simulink library "csc_sqt_sequential_trigger_mtv_lib"  (R2014b)
settings: Solver=ode45  SolverMode=SingleTasking  StartTime=0.0  StopTime=10.0  RelTol=1e-3
libraries: util_info_lib x1, csc_fcv_filter_convergence_lib x1, csc_squ_sequential_update_lib x1, csu_mmh_measurement_model_mtv_lib x1
settings Model: ExtModeAutoUpdateStatusClock=off  Creator=escrane  LastModifiedBy=mstewart

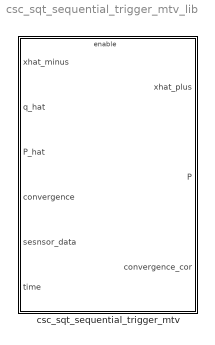
== system csc_sqt_sequential_trigger_mtv_lib ==
  csc_sqt_sequential_trigger_mtv : Subsystem  TreatAsAtomicUnit=on

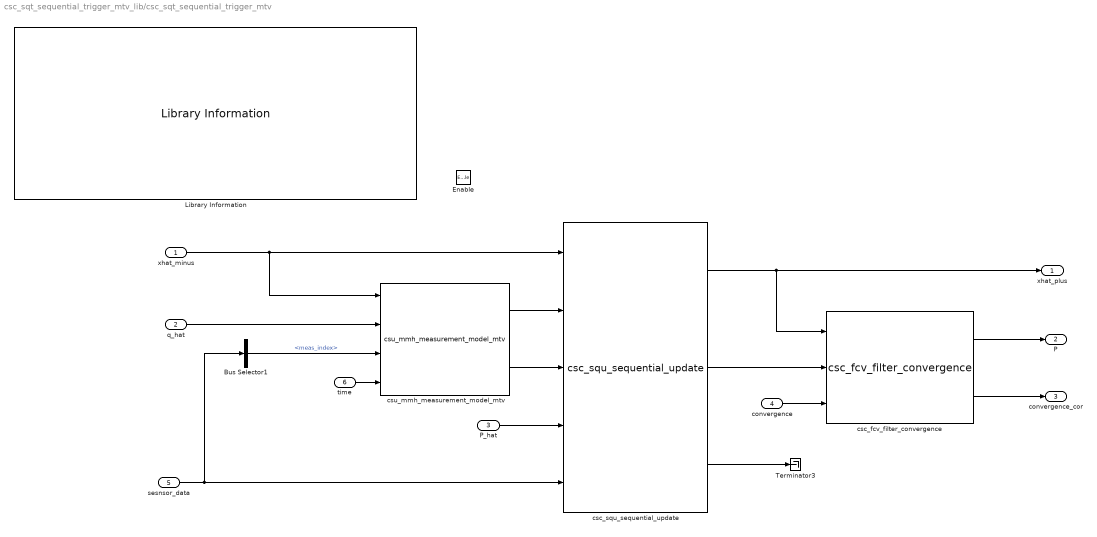
== system csc_sqt_sequential_trigger_mtv_lib/csc_sqt_sequential_trigger_mtv ==
  xhat_minus : Inport
  q_hat : Inport  Port=2
  P_hat : Inport  Port=3
  convergence : Inport  Port=4
  sesnsor_data : Inport  Port=5
  time : Inport  Port=6
  Enable : EnablePort
  Bus Selector1 : BusSelector  OutputSignals=meas_index
  Library Information : util_info_lib/Library Information  owner='NONE'
  Terminator3 : Terminator
  csc_fcv_filter_convergence : csc_fcv_filter_convergence_lib/csc_fcv_filter_convergence
  csc_squ_sequential_update : csc_squ_sequential_update_lib/csc_squ_sequential_update
  csu_mmh_measurement_model_mtv : csu_mmh_measurement_model_mtv_lib/csu_mmh_measurement_model_mtv
  xhat_plus : Outport
  P : Outport  Port=2
  convergence_cor : Outport  Port=3
  wires:
  convergence/1 -> csc_fcv_filter_convergence/3
  csc_squ_sequential_update/2 -> csc_fcv_filter_convergence/2
  csc_fcv_filter_convergence/2 -> convergence_cor/1
  csc_fcv_filter_convergence/1 -> P/1
  csc_squ_sequential_update/3 -> Terminator3/1
  time/1 -> csu_mmh_measurement_model_mtv/4
  csu_mmh_measurement_model_mtv/1 -> csc_squ_sequential_update/2
  Bus Selector1/1 -> csu_mmh_measurement_model_mtv/3  "<meas_index>"
  q_hat/1 -> csu_mmh_measurement_model_mtv/2
  csu_mmh_measurement_model_mtv/2 -> csc_squ_sequential_update/3
  xhat_minus/1 -> csc_squ_sequential_update/1, csu_mmh_measurement_model_mtv/1
  P_hat/1 -> csc_squ_sequential_update/4
  sesnsor_data/1 -> csc_squ_sequential_update/5, Bus Selector1/1
  csc_squ_sequential_update/1 -> xhat_plus/1, csc_fcv_filter_convergence/1
